simulink library "planar3linkslib"  (R2018a)
settings: Solver=VariableStepAuto  StartTime=0.0  StopTime=10.0  RelTol=1e-3
settings Model: Creator=corkep  LastModifiedBy=corkep

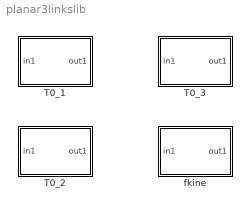
== system planar3linkslib ==
  T0_1 : MATLAB Function  TreatAsAtomicUnit=on
  T0_2 : MATLAB Function  TreatAsAtomicUnit=on
  T0_3 : MATLAB Function  TreatAsAtomicUnit=on
  fkine : MATLAB Function  TreatAsAtomicUnit=on

== matlab function planar3linkslib/T0_1 ==
  data: in1 input; out1 output
function out1 = T0_1(in1)
%#codegen

%    This function was generated by the Symbolic Math Toolbox version 8.1.
%    19-Aug-2018 15:04:10

q1 = in1(:,1);
t2 = cos(q1);
t3 = sin(q1);
out1 = reshape([t2,t3,0.0,0.0,-t3,t2,0.0,0.0,0.0,0.0,1.0,0.0,t2,t3,0.0,1.0],[4,4]);

== matlab function planar3linkslib/fkine ==
  data: in1 input; out1 output
function out1 = fkine(in1)
%#codegen

%    This function was generated by the Symbolic Math Toolbox version 8.1.
%    19-Aug-2018 15:04:10

q1 = in1(:,1);
q2 = in1(:,2);
q3 = in1(:,3);
t2 = q1+q2+q3;
t3 = cos(t2);
t4 = sin(t2);
t5 = q1+q2;
out1 = reshape([t3,t4,0.0,0.0,-t4,t3,0.0,0.0,0.0,0.0,1.0,0.0,t3+cos(q1)+cos(t5),t4+sin(q1)+sin(t5),0.0,1.0],[4,4]);

== matlab function planar3linkslib/T0_2 ==
  data: in1 input; out1 output
function out1 = T0_2(in1)
%#codegen

%    This function was generated by the Symbolic Math Toolbox version 8.1.
%    19-Aug-2018 15:04:11

q1 = in1(:,1);
q2 = in1(:,2);
t2 = cos(q1);
t3 = sin(q2);
t4 = cos(q2);
t5 = sin(q1);
t6 = t2.*t4;
t7 = t6-t3.*t5;
t8 = t2.*t3;
t9 = t4.*t5;
out1 = reshape([t7,t8+t9,0.0,0.0,-t2.*t3-t4.*t5,t7,0.0,0.0,0.0,0.0,1.0,0.0,t2+t6-t3.*t5,t5+t8+t9,0.0,1.0],[4,4]);

== matlab function planar3linkslib/T0_3 ==
  data: in1 input; out1 output
function out1 = T0_3(in1)
%#codegen

%    This function was generated by the Symbolic Math Toolbox version 8.1.
%    19-Aug-2018 15:04:11

q1 = in1(:,1);
q2 = in1(:,2);
q3 = in1(:,3);
t2 = cos(q1);
t3 = sin(q2);
t4 = cos(q2);
t5 = sin(q1);
t6 = cos(q3);
t7 = t2.*t3;
t8 = t4.*t5;
t9 = t7+t8;
t10 = sin(q3);
t11 = t2.*t4;
t13 = t3.*t5;
t12 = t11-t13;
t14 = t6.*t12;
t15 = t14-t9.*t10;
t16 = t6.*t9;
t17 = t10.*t12;
out1 = reshape([t15,t16+t17,0.0,0.0,-t6.*t9-t10.*t12,t15,0.0,0.0,0.0,0.0,1.0,0.0,t2+t11-t13+t14-t9.*t10,t5+t7+t8+t16+t17,0.0,1.0],[4,4]);
